simulink model "CodeGeneration"  (R2017a)
settings: Solver=VariableStepAuto  StartTime=0.0  StopTime=10.0  RelTol=1e-3
settings Model: Creator=Arthur  LastModifiedBy=Arthur

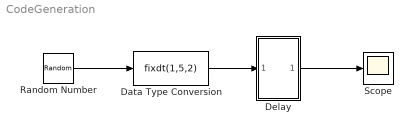
== system CodeGeneration ==
  Data Type Conversion : DataTypeConversion  OutDataTypeStr=fixdt(1,5,2)
  Delay : Subsystem
  Random Number : RandomNumber  SampleTime=0.1
  Scope : Scope
  wires:
  Random Number/1 -> Data Type Conversion/1
  Data Type Conversion/1 -> Delay/1(In1)
  Delay/1(Out1) -> Scope/1

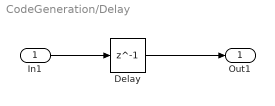
== system CodeGeneration/Delay ==
  In1 : Inport
  Delay : Delay  DelayLength=1
  Out1 : Outport
  wires:
  Delay/1 -> Out1/1
  In1/1 -> Delay/1
